simulink model "lab7"  (R2020a)
settings: Solver=FixedStepAuto  StartTime=0.0  StopTime=300  RelTol=1e-3
values from neighbouring files (symbols this model uses):
  a = max(abs(real([a1,a2])))    [pplane8.m]
  b = max(abs(imag([a1,a2])))    [pplane8.m]
  D = det(A)    [pplane8.m]
undefined symbols (not defined in the file or in its folder): A_2, g, h_bar, u_bar, u_max
settings Model: Creator=bruno  LastModifiedBy=bruno

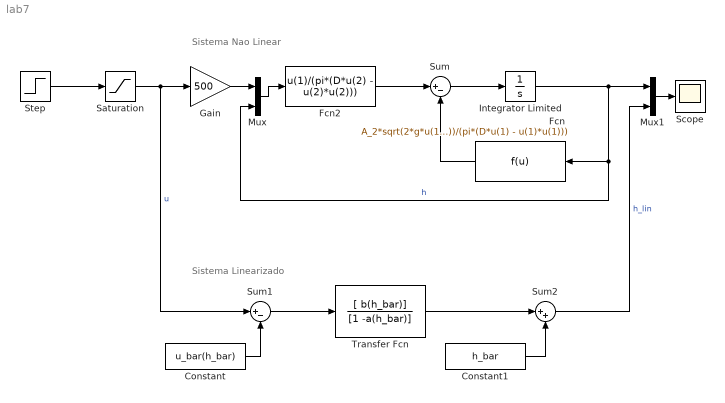
== system lab7 ==
  note: Sistema Linearizado
  note: Sistema Nao Linear
  Constant : Constant  Value=u_bar(h_bar)
  Constant1 : Constant  Value=h_bar
  Fcn : Fcn  Expr=A_2*sqrt(2*g*u(1))/(pi*(D*u(1) - u(1)*u(1)))
  Fcn2 : Fcn  Expr=u(1)/(pi*(D*u(2) - u(2)*u(2)))
  Gain : Gain  Gain=500
  Integrator Limited : Integrator  InitialCondition=h_bar  LimitOutput=on  UpperSaturationLimit=100-0.001  LowerSaturationLimit=0.001
  Mux : Mux  Inputs=2
  Mux1 : Mux  Inputs=2
  Saturation : Saturate  UpperLimit=u_max - 0.001  LowerLimit=0.001
  Scope : Scope
  Step : Step  Time=0  Before=u_bar(h_bar)  After=u_bar(h_bar) + 0.1  SampleTime=0
  Sum : Sum  Inputs=|+-
  Sum1 : Sum  Inputs=|+-
  Sum2 : Sum  Inputs=|++
  Transfer Fcn : TransferFcn  Numerator=[ b(h_bar)]  Denominator=[1 -a(h_bar)]
  wires:
  Sum/1 -> Integrator Limited/1
  Fcn2/1 -> Sum/1
  Fcn/1 -> Sum/2
  Saturation/1 -> Sum1/1, Gain/1  "u"
  Integrator Limited/1 -> Mux1/1, Fcn/1, Mux/2  "h"
  Step/1 -> Saturation/1
  Gain/1 -> Mux/1
  Mux/1 -> Fcn2/1
  Constant/1 -> Sum1/2
  Sum1/1 -> Transfer Fcn/1
  Constant1/1 -> Sum2/2
  Transfer Fcn/1 -> Sum2/1
  Mux1/1 -> Scope/1
  Sum2/1 -> Mux1/2  "h_lin"
